simulink subsystem "discrete_reduced_order_observer"  (R2024b)
settings: Solver=VariableStepAuto  StartTime=0.0  StopTime=10.0  RelTol=1e-3
values from neighbouring files (symbols this model uses):
  Gamma_o = [gamma2-L_obs*gamma1, (phi22-L_obs*phi12)*L_obs+phi21-L_obs*phi11]    [Controller_SS_direct_design_control_vars.m]
  H_o = [0;1]    [Controller_SS_direct_design_control_vars.m]
  J_o = [0, 1; 0, L_obs]    [Controller_SS_direct_design_control_vars.m]
  Phi_o = phi22 - L_obs * phi12    [Controller_SS_direct_design_control_vars.m]
  Ts = Ts_values(i)    [A_final_results.m]
settings Model: Creator=Riccardo Grosso  LastModifiedBy=Riccardo Grosso

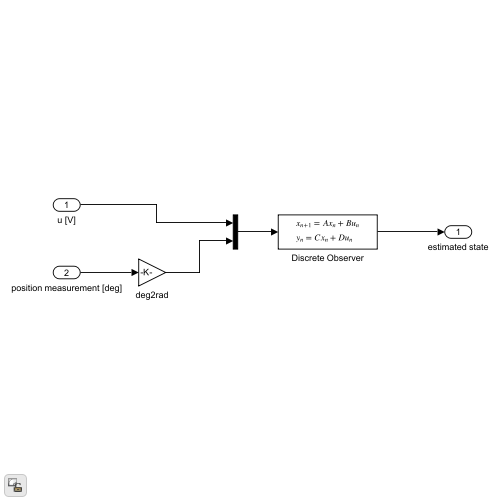
[thumbnail: Simulink's stored preview of the top-level diagram]
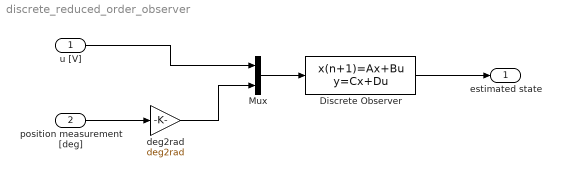
== system discrete_reduced_order_observer ==
  u [V] : Inport
  position measurement [deg] : Inport  Port=2
  Discrete Observer : DiscreteStateSpace  A=Phi_o  B=Gamma_o  C=H_o  D=J_o  SampleTime=Ts
  Mux : Mux  Inputs=2
  deg2rad : Gain  Gain=deg2rad
  estimated state : Outport
  wires:
  position measurement [deg]/1 -> deg2rad/1
  Mux/1 -> Discrete Observer/1
  u [V]/1 -> Mux/1
  deg2rad/1 -> Mux/2
  Discrete Observer/1 -> estimated state/1
